simulink model "SpringDamperinSimulink"  (R2019b)
settings: Solver=VariableStepAuto  StartTime=0.0  StopTime=10.0  RelTol=1e-3
values from neighbouring files (symbols this model uses):
  A = [0.7873 -0.3230;0.3230 0.7873]    [BarnsleyFern1.m]
  B = [0.0841 -0.3286;0.2930 0.0895]    [BarnsleyFern1.m]
  C = [-0.2458 0.1523;0.1722 0.3358]    [BarnsleyFern1.m]
undefined symbols (not defined in the file or in its folder): D, den, discr, num
settings Model: Creator=marslab  LastModifiedBy=marslab
settings DataIOCC: ReturnWorkspaceOutputs=off

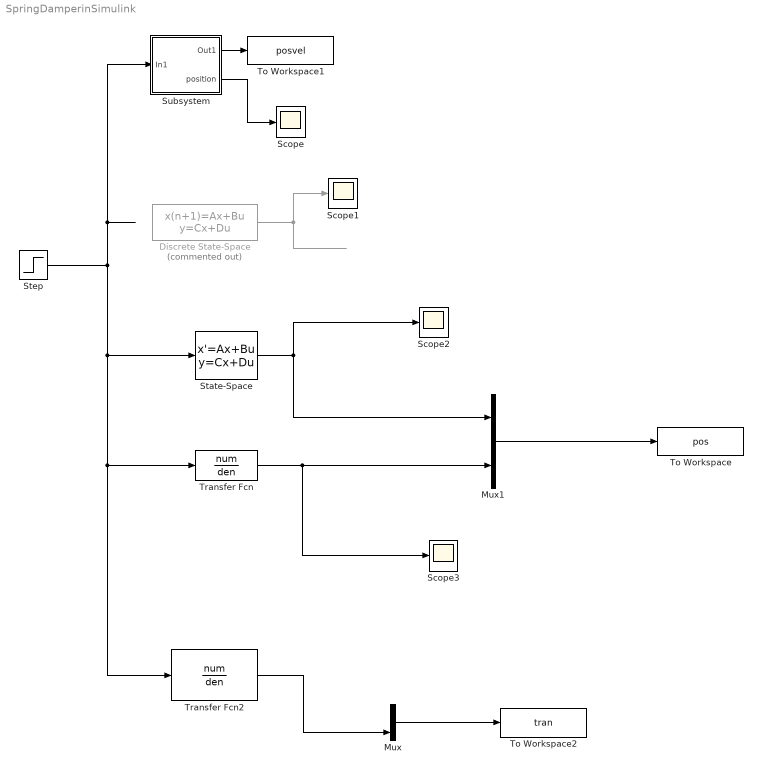
== system SpringDamperinSimulink ==
  Discrete State-Space : DiscreteStateSpace  Commented=on  A=discr.A  B=discr.B  C=discr.C  D=discr.D  SampleTime=0.1
  Mux : Mux  Inputs=2
  Mux1 : Mux  Inputs=2
  Scope{,1..3} (4 alike) : Scope
  State-Space : StateSpace  A=A  B=B  C=C  D=D  InitialCondition=0
  Step : Step  SampleTime=0.01
  Subsystem : Subsystem  mask{k=4, b=0.4}
      mask prompts: k "k="; b "b="
  To Workspace : ToWorkspace  VariableName=pos  SampleTime=-1
  To Workspace1 : ToWorkspace  VariableName=posvel  SampleTime=-1
  To Workspace2 : ToWorkspace  VariableName=tran  SampleTime=-1
  Transfer Fcn : TransferFcn  Numerator=num  Denominator=den
  Transfer Fcn2 : TransferFcn  Numerator=num  Denominator=den
  wires:
  Step/1 -> Transfer Fcn/1, Transfer Fcn2/1, State-Space/1, Subsystem/1(In1)
  Subsystem/1(Out1) -> To Workspace1/1
  Subsystem/2(position) -> Scope/1
  State-Space/1 -> Mux1/1, Scope2/1
  Transfer Fcn2/1 -> Mux/2
  Mux/1 -> To Workspace2/1
  Discrete State-Space/1 -> Scope1/1
  Mux1/1 -> To Workspace/1
  Transfer Fcn/1 -> Scope3/1, Mux1/2

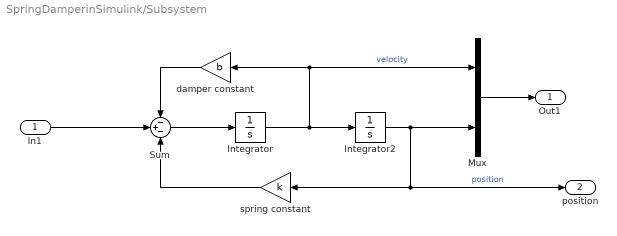
== system SpringDamperinSimulink/Subsystem ==
  In1 : Inport
  Integrator : Integrator
  Integrator2 : Integrator
  Mux : Mux  Inputs=2
  Sum : Sum  Inputs=-+-
  damper constant : Gain  Gain=b
  spring constant : Gain  Gain=k
  Out1 : Outport
  position : Outport  Port=2
  wires:
  Integrator2/1 -> Mux/2, position/1, spring constant/1  "position"
  damper constant/1 -> Sum/1
  Integrator/1 -> damper constant/1, Mux/1, Integrator2/1  "velocity"
  Sum/1 -> Integrator/1
  spring constant/1 -> Sum/3
  Mux/1 -> Out1/1
  In1/1 -> Sum/2
